simulink model "simple"  (Simulink 9.1)
settings: Solver=VariableStepAuto  StartTime=0.0  StopTime=10.0  RelTol=1e-3
settings Model: SuppressorTable=22 serialization::archive 11 0 6 0 0 0 1 0  Creator=wangjian  LastModifiedBy=wangjian
settings DataIOCC: SaveFormat=Dataset
settings OptimizationCC: LifeSpan=auto
settings DebuggingCC: UnderspecifiedInitializationDetection=Simplified  MergeDetectMultiDrivingBlocksExec=error  SFUnexpectedBacktrackingDiag=error  SFNoUnconditionalDefaultTransitionDiag=error  SFExecutionAtInitializationDiag=warning
settings HardwareCC: ProdBitPerPointer=64  ProdBitPerSizeT=64  ProdBitPerPtrDiffT=64  ProdLargestAtomicFloat=Float  ProdIntDivRoundTo=Zero  ProdEndianess=LittleEndian  ProdWordSize=64  ProdHWDeviceType=Intel->x86-64 (Windows64)
settings ModelReferenceCC: PropagateSignalLabelsOutOfModel=on
settings CodeAppCC: StateflowObjectComments=off
settings GRTTargetCC: TargetLangStandard=C99 (ISO)  CombineOutputUpdateFcns=on  GRTInterface=off
settings ConfigComp: CovMetricSettings=dwe  CovHtmlReporting=off  CovSaveCumulativeToWorkspaceVar=off  CovSaveSingleToWorkspaceVar=off  CovExternalEMLEnable=on

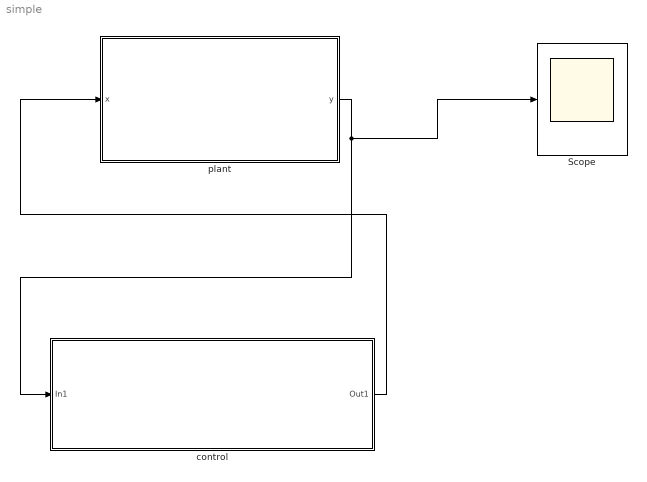
== system simple ==
  Scope : Scope
  control : Subsystem
  plant : Subsystem
  wires:
  plant/1(y) -> Scope/1, control/1(In1)
  control/1(Out1) -> plant/1(x)

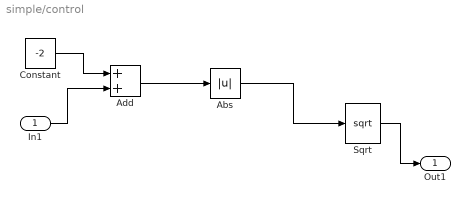
== system simple/control ==
  In1 : Inport
  Abs : Abs
  Add : Sum
  Constant : Constant  Value=-2
  Sqrt : Sqrt  SaturateOnIntegerOverflow=on
  Out1 : Outport
  wires:
  Constant/1 -> Add/1
  In1/1 -> Add/2
  Add/1 -> Abs/1
  Sqrt/1 -> Out1/1
  Abs/1 -> Sqrt/1

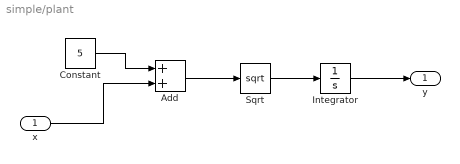
== system simple/plant ==
  x : Inport
  Add : Sum
  Constant : Constant  Value=5
  Integrator : Integrator
  Sqrt : Sqrt  SaturateOnIntegerOverflow=on
  y : Outport
  wires:
  x/1 -> Add/2
  Constant/1 -> Add/1
  Add/1 -> Sqrt/1
  Integrator/1 -> y/1
  Sqrt/1 -> Integrator/1
